simulink subsystem "vehicle_mdl"  (R2023a)
settings: Solver=VariableStepAuto  StartTime=0.0  StopTime=10.0  RelTol=1e-3
model mask{obj=obj}
  mask prompts: obj "Spring Object:"
settings Model: Creator=grouleau  LastModifiedBy=grouleau

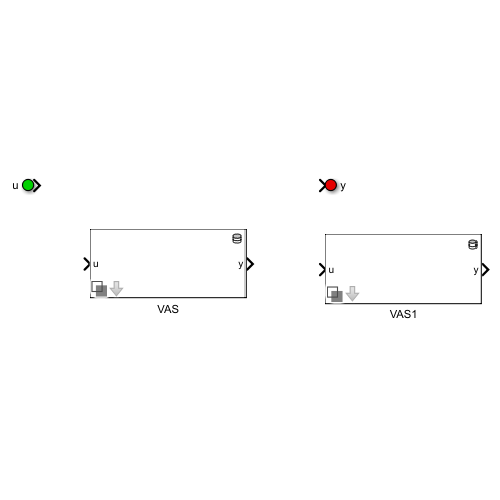
[thumbnail: Simulink's stored preview of the top-level diagram]
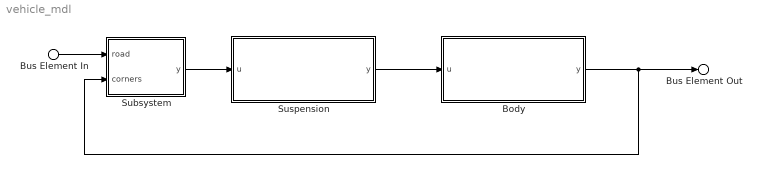
== system vehicle_mdl ==
  Bus Element In : Inport  PortName=u
  Body : Subsystem  Variant=on  VariantChoicesSpecifier=obj.getVariantChoices()  VariantControlMode=label  LabelModeActiveChoice=body_mdl  mask{obj=obj.Body}
      mask prompts: obj "Part Object"
  Subsystem : Subsystem
  Suspension : Subsystem  Variant=on  VariantChoicesSpecifier=obj.getVariantChoices()  VariantControlMode=label  LabelModeActiveChoice=suspensionThreeDOF  mask{obj=obj.Suspension}
      mask prompts: obj "Part Object"
  Bus Element Out : Outport  PortName=y
  wires:
  Body/1(y) -> Bus Element Out/1, Subsystem/2(corners)
  Suspension/1(y) -> Body/1(u)
  Bus Element In/1 -> Subsystem/1(road)
  Subsystem/1(y) -> Suspension/1(u)

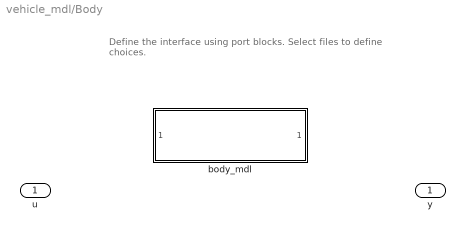
== system vehicle_mdl/Body ==
  note: Define the interface using port blocks.
      | Select files to define choices.
  u : Inport
  body_mdl : Subsystem  VariantControl=body_mdl  ReferencedSubsystem=body_mdl  obj=obj
  y : Outport

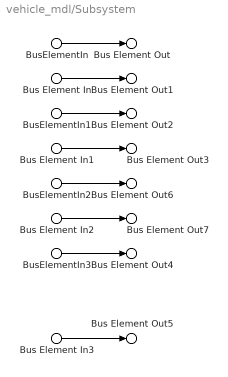
== system vehicle_mdl/Subsystem ==
  Bus Element In : Inport  PortName=road  Element=FrontLeft
  Bus Element In1 : Inport  PortName=road  Element=FrontLeft
  Bus Element In2 : Inport  PortName=road  Element=RearLeft
  Bus Element In3 : Inport  PortName=road  Element=RearRight
  BusElementIn : Inport  Port=2  PortName=corners  Element=FrontLeft
  BusElementIn1 : Inport  Port=2  PortName=corners  Element=FrontRight
  BusElementIn2 : Inport  Port=2  PortName=corners  Element=RearLeft
  BusElementIn3 : Inport  Port=2  PortName=corners  Element=RearRight
  Bus Element Out2 : Outport  PortName=y  Element=FrontRight.body
  Bus Element Out3 : Outport  PortName=y  Element=FrontRight.road
  Bus Element Out : Outport  PortName=y  Element=FrontLeft.body
  Bus Element Out1 : Outport  PortName=y  Element=FrontLeft.road
  Bus Element Out6 : Outport  PortName=y  Element=RearLeft.body
  Bus Element Out7 : Outport  PortName=y  Element=RearLeft.road
  Bus Element Out4 : Outport  PortName=y  Element=RearRight.body
  Bus Element Out5 : Outport  PortName=y  Element=RearRight.road
  wires:
  BusElementIn2/1 -> Bus Element Out6/1
  Bus Element In2/1 -> Bus Element Out7/1
  Bus Element In3/1 -> Bus Element Out5/1
  BusElementIn3/1 -> Bus Element Out4/1
  BusElementIn1/1 -> Bus Element Out2/1
  Bus Element In1/1 -> Bus Element Out3/1
  Bus Element In/1 -> Bus Element Out1/1
  BusElementIn/1 -> Bus Element Out/1

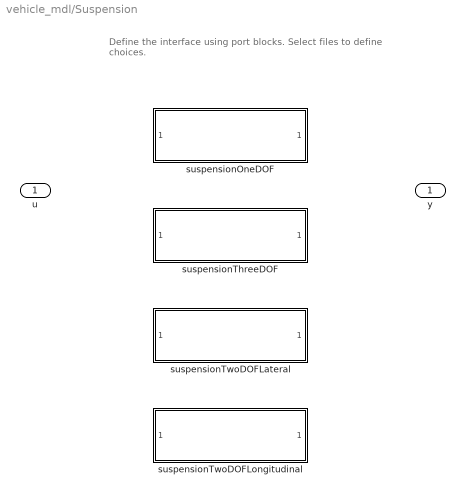
== system vehicle_mdl/Suspension ==
  note: Define the interface using port blocks.
      | Select files to define choices.
  u : Inport
  suspensionOneDOF : Subsystem  VariantControl=suspensionOneDOF  ReferencedSubsystem=suspensionOneDOF  obj=obj
  suspensionThreeDOF : Subsystem  VariantControl=suspensionThreeDOF  ReferencedSubsystem=suspensionThreeDOF  obj=obj
  suspensionTwoDOFLateral : Subsystem  VariantControl=suspensionTwoDOFLateral  ReferencedSubsystem=suspensionTwoDOFLateral  obj=obj
  suspensionTwoDOFLongitudinal : Subsystem  VariantControl=suspensionTwoDOFLongitudinal  ReferencedSubsystem=suspensionTwoDOFLongitudinal  obj=obj
  y : Outport
